simulink model "Alpha_Architecture"  (R2020b)
settings: Solver=VariableStepAuto  StartTime=0.0  StopTime=10.0  RelTol=1e-3
settings Model: DataDictionary=Alpha_ArchitectureDD_1.sldd  OrderedModelArguments=off  Creator=Josh_  LastModifiedBy=jbmic

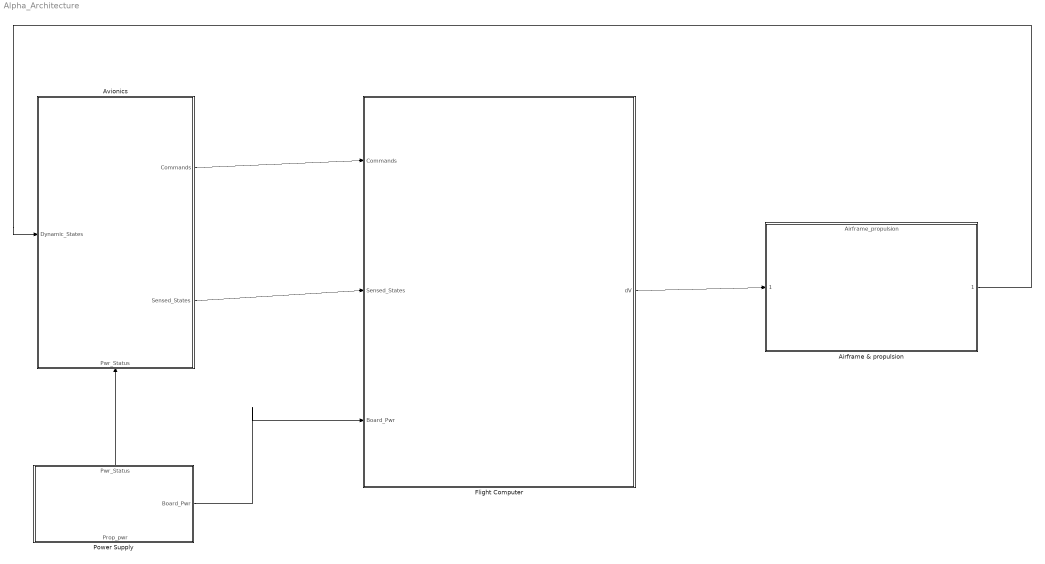
== system Alpha_Architecture ==
  Airframe & propulsion : ModelReference  ModelNameDialog=Airframe_propulsion  SimulationMode=Normal  ModelReferenceVersion=1.6
      settings: PortSchema="{\"entries\":[{\"content\":{\"headerSize\":38,\"margin\":15,\"minimumSpacing\":25,\"sides\":[{\"content\":{\"connectorIds\":[\"In1\"]},\"type\":\"ConnectorPlacement.EquallySpacedRectSide\",\"uuid\":\"5a96790b-1a4b-40de-9237-fa3ed351c29d\"},{\"content\":{\"connectorIds\":[\"Out1\"],\"side\":\"RIGHT\"},\"type\":\"ConnectorPlacement.EquallySpacedRectSide\",\"uuid\":\"65d1e4af-73af-4bc2-af7a-5ddd32d587af\"},{\"content\":{\"connectorIds\":[],\"side\":\"TOP\"},\"type\":\"ConnectorPlacement.EquallySpacedRectSide\",\"uuid\":\"28da9753-bb87-4f53-bc0d-c389ea44753a\"},{\"content\":{\"connectorIds\":[],\"side\":\"HIDDEN\"},\"type\":\"ConnectorPlacement.EquallySpacedRectSide\",\"uuid\":\"87ff2825-dc0e-4fcc-9b37-401c5c54474f\"}]},\"type\":\"ConnectorPlacement.EquallySpacedConnector\",\"uuid\":\"52ab39f8-c1eb-4e75-9fe9-b0e1857d3d38\"}],\"packageUris\":[\"http://schema.mathworks.com/mf0/Connector/R2020b\"],\"version\":\"1.0\"}"
  Avionics : Subsystem
      settings: PortSchema="{\"entries\":[{\"content\":{\"headerSize\":26,\"margin\":15,\"minimumSpacing\":25,\"sides\":[{\"content\":{\"connectorIds\":[\"In1\"]},\"type\":\"ConnectorPlacement.EquallySpacedRectSide\",\"uuid\":\"f0eb9bf2-bfee-4043-a89e-343ddad828c0\"},{\"content\":{\"connectorIds\":[\"Out1\",\"Out2\"],\"side\":\"RIGHT\"},\"type\":\"ConnectorPlacement.EquallySpacedRectSide\",\"uuid\":\"59a31ab0-f936-4a77-903b-0592fc94f50c\"},{\"content\":{\"connectorIds\":[],\"side\":\"TOP\"},\"type\":\"ConnectorPlacement.EquallySpacedRectSide\",\"uuid\":\"00c9f7f6-e065-44bb-91eb-10654e948fa4\"},{\"content\":{\"connectorIds\":[\"In2\"],\"side\":\"BOTTOM\"},\"type\":\"ConnectorPlacement.EquallySpacedRectSide\",\"uuid\":\"1c3b996c-1062-4d5b-bb11-b7de8dcf6a0a\"},{\"content\":{\"connectorIds\":[],\"side\":\"HIDDEN\"},\"type\":\"ConnectorPlacement.EquallySpacedRectSide\",\"uuid\":\"997c3d97-1a3e-4a81-af6b-83f3ee2d82f5\"}]},\"type\":\"ConnectorPlacement.EquallySpacedConnector\",\"uuid\":\"01157a40-eaa9-4a5a-9ab5-20d6af6643e5\"}],\"packageUris\":[\"http://schema.mathworks.com/mf0/Connector/R2020b\"],\"version\":\"1.0\"}"
  Flight Computer : Subsystem
      settings: PortSchema="{\"entries\":[{\"content\":{\"headerSize\":26,\"margin\":15,\"minimumSpacing\":25,\"sides\":[{\"content\":{\"connectorIds\":[\"In1\",\"In3\",\"In2\"]},\"type\":\"ConnectorPlacement.EquallySpacedRectSide\",\"uuid\":\"f0eb9bf2-bfee-4043-a89e-343ddad828c0\"},{\"content\":{\"connectorIds\":[\"Out1\"],\"side\":\"RIGHT\"},\"type\":\"ConnectorPlacement.EquallySpacedRectSide\",\"uuid\":\"59a31ab0-f936-4a77-903b-0592fc94f50c\"},{\"content\":{\"connectorIds\":[],\"side\":\"TOP\"},\"type\":\"ConnectorPlacement.EquallySpacedRectSide\",\"uuid\":\"00c9f7f6-e065-44bb-91eb-10654e948fa4\"},{\"content\":{\"connectorIds\":[],\"side\":\"BOTTOM\"},\"type\":\"ConnectorPlacement.EquallySpacedRectSide\",\"uuid\":\"e1a67c33-68ba-4a6b-a9bd-5a291173929b\"},{\"content\":{\"connectorIds\":[],\"side\":\"HIDDEN\"},\"type\":\"ConnectorPlacement.EquallySpacedRectSide\",\"uuid\":\"997c3d97-1a3e-4a81-af6b-83f3ee2d82f5\"}]},\"type\":\"ConnectorPlacement.EquallySpacedConnector\",\"uuid\":\"01157a40-eaa9-4a5a-9ab5-20d6af6643e5\"}],\"packageUris\":[\"http://schema.mathworks.com/mf0/Connector/R2020b\"],\"version\":\"1.0\"}"
  Power Supply : Subsystem
      settings: PortSchema="{\"entries\":[{\"content\":{\"headerSize\":26,\"margin\":15,\"minimumSpacing\":25,\"sides\":[{\"content\":{\"connectorIds\":[]},\"type\":\"ConnectorPlacement.EquallySpacedRectSide\",\"uuid\":\"f0eb9bf2-bfee-4043-a89e-343ddad828c0\"},{\"content\":{\"connectorIds\":[\"Out1\"],\"side\":\"RIGHT\"},\"type\":\"ConnectorPlacement.EquallySpacedRectSide\",\"uuid\":\"59a31ab0-f936-4a77-903b-0592fc94f50c\"},{\"content\":{\"connectorIds\":[\"Out3\"],\"side\":\"TOP\"},\"type\":\"ConnectorPlacement.EquallySpacedRectSide\",\"uuid\":\"00c9f7f6-e065-44bb-91eb-10654e948fa4\"},{\"content\":{\"connectorIds\":[\"Out2\"],\"side\":\"BOTTOM\"},\"type\":\"ConnectorPlacement.EquallySpacedRectSide\",\"uuid\":\"a7244861-68c9-40bc-a682-7b968120676e\"},{\"content\":{\"connectorIds\":[],\"side\":\"HIDDEN\"},\"type\":\"ConnectorPlacement.EquallySpacedRectSide\",\"uuid\":\"997c3d97-1a3e-4a81-af6b-83f3ee2d82f5\"}]},\"type\":\"ConnectorPlacement.EquallySpacedConnector\",\"uuid\":\"01157a40-eaa9-4a5a-9ab5-20d6af6643e5\"}],\"packageUris\":[\"http://schema.mathworks.com/mf0/Connector/R2020b\"],\"version\":\"1.0\"}"
  wires:
  Avionics/2(Sensed_States) -> Flight Computer/3(Sensed_States)
  Power Supply/3(Pwr_Status) -> Avionics/2(Pwr_Status)
  Avionics/1(Commands) -> Flight Computer/1(Commands)
  Power Supply/1(Board_Pwr) -> Flight Computer/2(Board_Pwr)
  Flight Computer/1(dV) -> Airframe & propulsion/1
  Airframe & propulsion/1 -> Avionics/1(Dynamic_States)

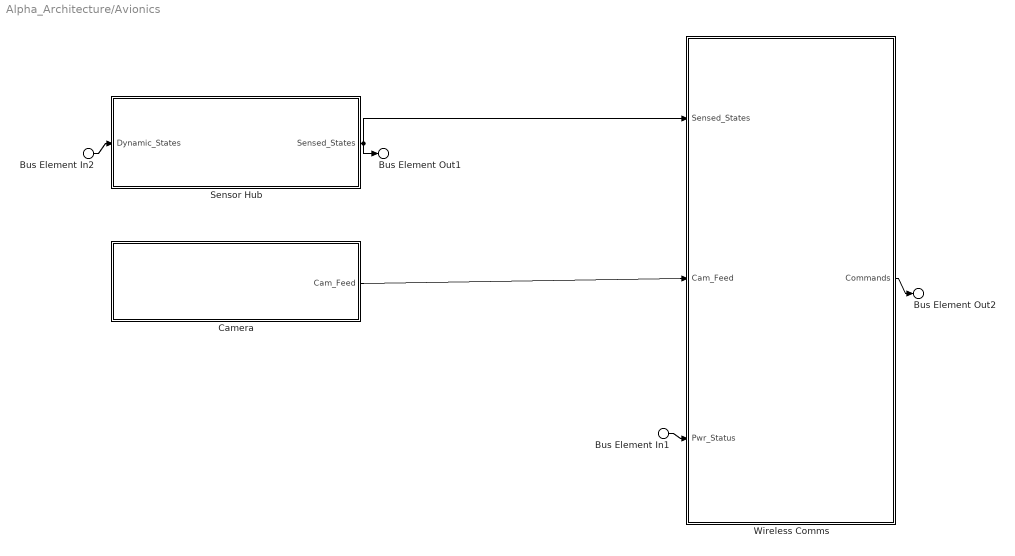
== system Alpha_Architecture/Avionics ==
  Bus Element In2 : Inport  PortName=Dynamic_States
  Bus Element In1 : Inport  Port=2  PortName=Pwr_Status
  Camera : Subsystem
      settings: PortSchema="{\"entries\":[{\"content\":{\"headerSize\":26,\"margin\":15,\"minimumSpacing\":25,\"sides\":[{\"content\":{\"connectorIds\":[]},\"type\":\"ConnectorPlacement.EquallySpacedRectSide\",\"uuid\":\"f0eb9bf2-bfee-4043-a89e-343ddad828c0\"},{\"content\":{\"connectorIds\":[\"Out1\"],\"side\":\"RIGHT\"},\"type\":\"ConnectorPlacement.EquallySpacedRectSide\",\"uuid\":\"59a31ab0-f936-4a77-903b-0592fc94f50c\"},{\"content\":{\"connectorIds\":[],\"side\":\"TOP\"},\"type\":\"ConnectorPlacement.EquallySpacedRectSide\",\"uuid\":\"00c9f7f6-e065-44bb-91eb-10654e948fa4\"},{\"content\":{\"connectorIds\":[],\"side\":\"HIDDEN\"},\"type\":\"ConnectorPlacement.EquallySpacedRectSide\",\"uuid\":\"997c3d97-1a3e-4a81-af6b-83f3ee2d82f5\"}]},\"type\":\"ConnectorPlacement.EquallySpacedConnector\",\"uuid\":\"01157a40-eaa9-4a5a-9ab5-20d6af6643e5\"}],\"packageUris\":[\"http://schema.mathworks.com/mf0/Connector/R2020b\"],\"version\":\"1.0\"}"
  Sensor Hub : Subsystem
      settings: PortSchema="{\"entries\":[{\"content\":{\"headerSize\":26,\"margin\":15,\"minimumSpacing\":25,\"sides\":[{\"content\":{\"connectorIds\":[\"In1\"]},\"type\":\"ConnectorPlacement.EquallySpacedRectSide\",\"uuid\":\"f0eb9bf2-bfee-4043-a89e-343ddad828c0\"},{\"content\":{\"connectorIds\":[\"Out1\"],\"side\":\"RIGHT\"},\"type\":\"ConnectorPlacement.EquallySpacedRectSide\",\"uuid\":\"59a31ab0-f936-4a77-903b-0592fc94f50c\"},{\"content\":{\"connectorIds\":[],\"side\":\"TOP\"},\"type\":\"ConnectorPlacement.EquallySpacedRectSide\",\"uuid\":\"00c9f7f6-e065-44bb-91eb-10654e948fa4\"},{\"content\":{\"connectorIds\":[],\"side\":\"HIDDEN\"},\"type\":\"ConnectorPlacement.EquallySpacedRectSide\",\"uuid\":\"997c3d97-1a3e-4a81-af6b-83f3ee2d82f5\"}]},\"type\":\"ConnectorPlacement.EquallySpacedConnector\",\"uuid\":\"01157a40-eaa9-4a5a-9ab5-20d6af6643e5\"}],\"packageUris\":[\"http://schema.mathworks.com/mf0/Connector/R2020b\"],\"version\":\"1.0\"}"
  Wireless Comms : Subsystem
      settings: PortSchema="{\"entries\":[{\"content\":{\"headerSize\":26,\"margin\":15,\"minimumSpacing\":25,\"sides\":[{\"content\":{\"connectorIds\":[\"In3\",\"In2\",\"In1\"]},\"type\":\"ConnectorPlacement.EquallySpacedRectSide\",\"uuid\":\"f0eb9bf2-bfee-4043-a89e-343ddad828c0\"},{\"content\":{\"connectorIds\":[\"Out1\"],\"side\":\"RIGHT\"},\"type\":\"ConnectorPlacement.EquallySpacedRectSide\",\"uuid\":\"59a31ab0-f936-4a77-903b-0592fc94f50c\"},{\"content\":{\"connectorIds\":[],\"side\":\"TOP\"},\"type\":\"ConnectorPlacement.EquallySpacedRectSide\",\"uuid\":\"00c9f7f6-e065-44bb-91eb-10654e948fa4\"},{\"content\":{\"connectorIds\":[],\"side\":\"HIDDEN\"},\"type\":\"ConnectorPlacement.EquallySpacedRectSide\",\"uuid\":\"997c3d97-1a3e-4a81-af6b-83f3ee2d82f5\"}]},\"type\":\"ConnectorPlacement.EquallySpacedConnector\",\"uuid\":\"01157a40-eaa9-4a5a-9ab5-20d6af6643e5\"}],\"packageUris\":[\"http://schema.mathworks.com/mf0/Connector/R2020b\"],\"version\":\"1.0\"}"
  Bus Element Out2 : Outport  PortName=Commands
  Bus Element Out1 : Outport  Port=2  PortName=Sensed_States
  wires:
  Camera/1(Cam_Feed) -> Wireless Comms/2(Cam_Feed)
  Sensor Hub/1(Sensed_States) -> Wireless Comms/3(Sensed_States), Bus Element Out1/1
  Bus Element In1/1 -> Wireless Comms/1(Pwr_Status)
  Wireless Comms/1(Commands) -> Bus Element Out2/1
  Bus Element In2/1 -> Sensor Hub/1(Dynamic_States)

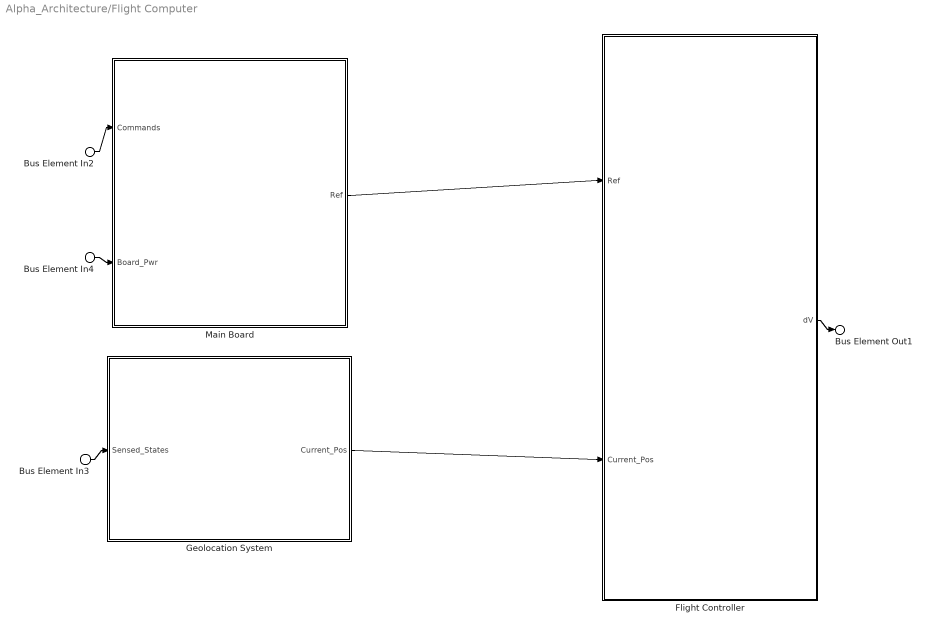
== system Alpha_Architecture/Flight Computer ==
  Bus Element In2 : Inport  PortName=Commands
  Bus Element In4 : Inport  Port=2  PortName=Board_Pwr
  Bus Element In3 : Inport  Port=3  PortName=Sensed_States
  Flight Controller : Subsystem
      settings: PortSchema="{\"entries\":[{\"content\":{\"headerSize\":26,\"margin\":15,\"minimumSpacing\":25,\"sides\":[{\"content\":{\"connectorIds\":[\"In1\",\"In2\"]},\"type\":\"ConnectorPlacement.EquallySpacedRectSide\",\"uuid\":\"f0eb9bf2-bfee-4043-a89e-343ddad828c0\"},{\"content\":{\"connectorIds\":[\"Out1\"],\"side\":\"RIGHT\"},\"type\":\"ConnectorPlacement.EquallySpacedRectSide\",\"uuid\":\"59a31ab0-f936-4a77-903b-0592fc94f50c\"},{\"content\":{\"connectorIds\":[],\"side\":\"TOP\"},\"type\":\"ConnectorPlacement.EquallySpacedRectSide\",\"uuid\":\"00c9f7f6-e065-44bb-91eb-10654e948fa4\"},{\"content\":{\"connectorIds\":[],\"side\":\"BOTTOM\"},\"type\":\"ConnectorPlacement.EquallySpacedRectSide\",\"uuid\":\"961fc88a-8781-4ec4-8a6a-b42b081babd4\"},{\"content\":{\"connectorIds\":[],\"side\":\"HIDDEN\"},\"type\":\"ConnectorPlacement.EquallySpacedRectSide\",\"uuid\":\"997c3d97-1a3e-4a81-af6b-83f3ee2d82f5\"}]},\"type\":\"ConnectorPlacement.EquallySpacedConnector\",\"uuid\":\"01157a40-eaa9-4a5a-9ab5-20d6af6643e5\"}],\"packageUris\":[\"http://schema.mathworks.com/mf0/Connector/R2020b\"],\"version\":\"1.0\"}"
  Geolocation System : Subsystem
      settings: PortSchema="{\"entries\":[{\"content\":{\"headerSize\":26,\"margin\":15,\"minimumSpacing\":25,\"sides\":[{\"content\":{\"connectorIds\":[\"In1\"]},\"type\":\"ConnectorPlacement.EquallySpacedRectSide\",\"uuid\":\"f0eb9bf2-bfee-4043-a89e-343ddad828c0\"},{\"content\":{\"connectorIds\":[\"Out1\"],\"side\":\"RIGHT\"},\"type\":\"ConnectorPlacement.EquallySpacedRectSide\",\"uuid\":\"59a31ab0-f936-4a77-903b-0592fc94f50c\"},{\"content\":{\"connectorIds\":[],\"side\":\"TOP\"},\"type\":\"ConnectorPlacement.EquallySpacedRectSide\",\"uuid\":\"00c9f7f6-e065-44bb-91eb-10654e948fa4\"},{\"content\":{\"connectorIds\":[],\"side\":\"HIDDEN\"},\"type\":\"ConnectorPlacement.EquallySpacedRectSide\",\"uuid\":\"997c3d97-1a3e-4a81-af6b-83f3ee2d82f5\"}]},\"type\":\"ConnectorPlacement.EquallySpacedConnector\",\"uuid\":\"01157a40-eaa9-4a5a-9ab5-20d6af6643e5\"}],\"packageUris\":[\"http://schema.mathworks.com/mf0/Connector/R2020b\"],\"version\":\"1.0\"}"
  Main Board : Subsystem
      settings: PortSchema="{\"entries\":[{\"content\":{\"headerSize\":26,\"margin\":15,\"minimumSpacing\":25,\"sides\":[{\"content\":{\"connectorIds\":[\"In2\",\"In1\"]},\"type\":\"ConnectorPlacement.EquallySpacedRectSide\",\"uuid\":\"f0eb9bf2-bfee-4043-a89e-343ddad828c0\"},{\"content\":{\"connectorIds\":[\"Out1\"],\"side\":\"RIGHT\"},\"type\":\"ConnectorPlacement.EquallySpacedRectSide\",\"uuid\":\"59a31ab0-f936-4a77-903b-0592fc94f50c\"},{\"content\":{\"connectorIds\":[],\"side\":\"TOP\"},\"type\":\"ConnectorPlacement.EquallySpacedRectSide\",\"uuid\":\"00c9f7f6-e065-44bb-91eb-10654e948fa4\"},{\"content\":{\"connectorIds\":[],\"side\":\"BOTTOM\"},\"type\":\"ConnectorPlacement.EquallySpacedRectSide\",\"uuid\":\"d3df3a47-29ff-4127-ba11-03dc604beefc\"},{\"content\":{\"connectorIds\":[],\"side\":\"HIDDEN\"},\"type\":\"ConnectorPlacement.EquallySpacedRectSide\",\"uuid\":\"997c3d97-1a3e-4a81-af6b-83f3ee2d82f5\"}]},\"type\":\"ConnectorPlacement.EquallySpacedConnector\",\"uuid\":\"01157a40-eaa9-4a5a-9ab5-20d6af6643e5\"}],\"packageUris\":[\"http://schema.mathworks.com/mf0/Connector/R2020b\"],\"version\":\"1.0\"}"
  Bus Element Out1 : Outport  PortName=dV
  wires:
  Flight Controller/1(dV) -> Bus Element Out1/1
  Main Board/1(Ref) -> Flight Controller/1(Ref)
  Bus Element In2/1 -> Main Board/2(Commands)
  Bus Element In4/1 -> Main Board/1(Board_Pwr)
  Bus Element In3/1 -> Geolocation System/1(Sensed_States)
  Geolocation System/1(Current_Pos) -> Flight Controller/2(Current_Pos)

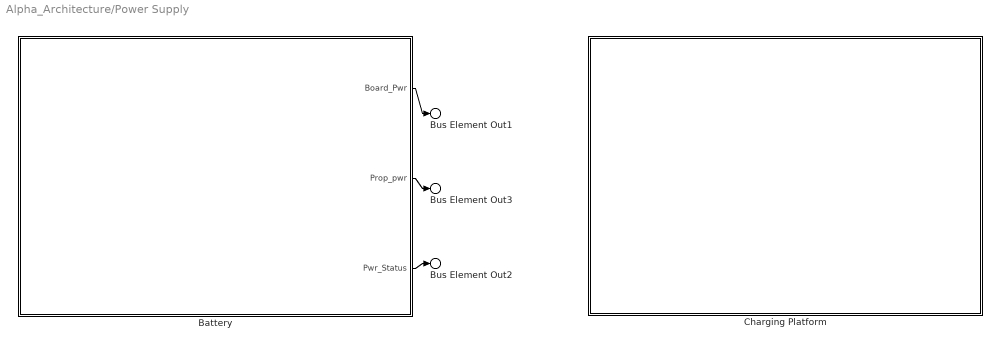
== system Alpha_Architecture/Power Supply ==
  Battery : Subsystem
      settings: PortSchema="{\"entries\":[{\"content\":{\"headerSize\":26,\"margin\":15,\"minimumSpacing\":25,\"sides\":[{\"content\":{\"connectorIds\":[]},\"type\":\"ConnectorPlacement.EquallySpacedRectSide\",\"uuid\":\"f0eb9bf2-bfee-4043-a89e-343ddad828c0\"},{\"content\":{\"connectorIds\":[\"Out1\",\"Out2\",\"Out3\"],\"side\":\"RIGHT\"},\"type\":\"ConnectorPlacement.EquallySpacedRectSide\",\"uuid\":\"59a31ab0-f936-4a77-903b-0592fc94f50c\"},{\"content\":{\"connectorIds\":[],\"side\":\"TOP\"},\"type\":\"ConnectorPlacement.EquallySpacedRectSide\",\"uuid\":\"00c9f7f6-e065-44bb-91eb-10654e948fa4\"},{\"content\":{\"connectorIds\":[],\"side\":\"HIDDEN\"},\"type\":\"ConnectorPlacement.EquallySpacedRectSide\",\"uuid\":\"997c3d97-1a3e-4a81-af6b-83f3ee2d82f5\"}]},\"type\":\"ConnectorPlacement.EquallySpacedConnector\",\"uuid\":\"01157a40-eaa9-4a5a-9ab5-20d6af6643e5\"}],\"packageUris\":[\"http://schema.mathworks.com/mf0/Connector/R2020b\"],\"version\":\"1.0\"}"
  Charging Platform : Subsystem
      settings: PortSchema="{\"entries\":[{\"content\":{\"headerSize\":26,\"margin\":15,\"minimumSpacing\":25,\"sides\":[{\"content\":{\"connectorIds\":[]},\"type\":\"ConnectorPlacement.EquallySpacedRectSide\",\"uuid\":\"f0eb9bf2-bfee-4043-a89e-343ddad828c0\"},{\"content\":{\"connectorIds\":[],\"side\":\"RIGHT\"},\"type\":\"ConnectorPlacement.EquallySpacedRectSide\",\"uuid\":\"59a31ab0-f936-4a77-903b-0592fc94f50c\"},{\"content\":{\"connectorIds\":[],\"side\":\"TOP\"},\"type\":\"ConnectorPlacement.EquallySpacedRectSide\",\"uuid\":\"00c9f7f6-e065-44bb-91eb-10654e948fa4\"},{\"content\":{\"connectorIds\":[],\"side\":\"HIDDEN\"},\"type\":\"ConnectorPlacement.EquallySpacedRectSide\",\"uuid\":\"997c3d97-1a3e-4a81-af6b-83f3ee2d82f5\"}]},\"type\":\"ConnectorPlacement.EquallySpacedConnector\",\"uuid\":\"01157a40-eaa9-4a5a-9ab5-20d6af6643e5\"}],\"packageUris\":[\"http://schema.mathworks.com/mf0/Connector/R2020b\"],\"version\":\"1.0\"}"
  Bus Element Out1 : Outport  PortName=Board_Pwr
  Bus Element Out3 : Outport  Port=2  PortName=Prop_pwr
  Bus Element Out2 : Outport  Port=3  PortName=Pwr_Status
  wires:
  Battery/3(Pwr_Status) -> Bus Element Out2/1
  Battery/1(Board_Pwr) -> Bus Element Out1/1
  Battery/2(Prop_pwr) -> Bus Element Out3/1

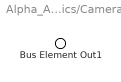
== system Alpha_Architecture/Avionics/Camera ==
  Bus Element Out1 : Outport  PortName=Cam_Feed

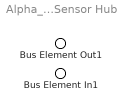
== system Alpha_Architecture/Avionics/Sensor Hub ==
  Bus Element In1 : Inport  PortName=Dynamic_States
  Bus Element Out1 : Outport  PortName=Sensed_States

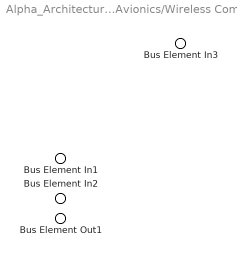
== system Alpha_Architecture/Avionics/Wireless Comms ==
  Bus Element In3 : Inport  PortName=Pwr_Status
  Bus Element In1 : Inport  Port=2  PortName=Cam_Feed
  Bus Element In2 : Inport  Port=3  PortName=Sensed_States
  Bus Element Out1 : Outport  PortName=Commands

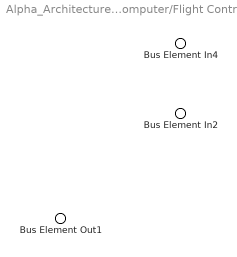
== system Alpha_Architecture/Flight Computer/Flight Controller ==
  Bus Element In4 : Inport  PortName=Ref
  Bus Element In2 : Inport  Port=2  PortName=Current_Pos
  Bus Element Out1 : Outport  PortName=dV

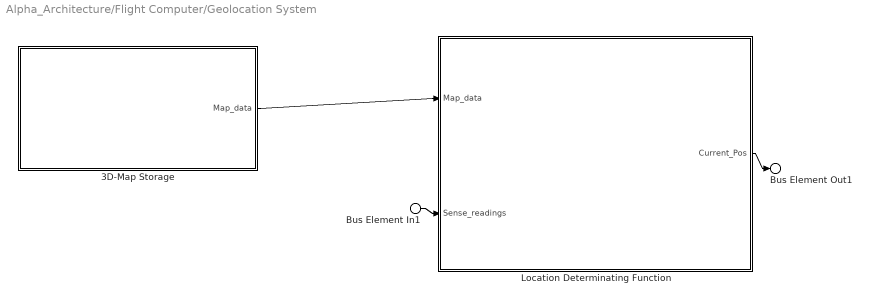
== system Alpha_Architecture/Flight Computer/Geolocation System ==
  Bus Element In1 : Inport  PortName=Sensed_States
  3D-Map Storage : Subsystem
      settings: PortSchema="{\"entries\":[{\"content\":{\"headerSize\":26,\"margin\":15,\"minimumSpacing\":25,\"sides\":[{\"content\":{\"connectorIds\":[]},\"type\":\"ConnectorPlacement.EquallySpacedRectSide\",\"uuid\":\"f0eb9bf2-bfee-4043-a89e-343ddad828c0\"},{\"content\":{\"connectorIds\":[\"Out1\"],\"side\":\"RIGHT\"},\"type\":\"ConnectorPlacement.EquallySpacedRectSide\",\"uuid\":\"59a31ab0-f936-4a77-903b-0592fc94f50c\"},{\"content\":{\"connectorIds\":[],\"side\":\"TOP\"},\"type\":\"ConnectorPlacement.EquallySpacedRectSide\",\"uuid\":\"00c9f7f6-e065-44bb-91eb-10654e948fa4\"},{\"content\":{\"connectorIds\":[],\"side\":\"HIDDEN\"},\"type\":\"ConnectorPlacement.EquallySpacedRectSide\",\"uuid\":\"997c3d97-1a3e-4a81-af6b-83f3ee2d82f5\"}]},\"type\":\"ConnectorPlacement.EquallySpacedConnector\",\"uuid\":\"01157a40-eaa9-4a5a-9ab5-20d6af6643e5\"}],\"packageUris\":[\"http://schema.mathworks.com/mf0/Connector/R2020b\"],\"version\":\"1.0\"}"
  Location Determinating Function : Subsystem
      settings: PortSchema="{\"entries\":[{\"content\":{\"headerSize\":26,\"margin\":15,\"minimumSpacing\":25,\"sides\":[{\"content\":{\"connectorIds\":[\"In1\",\"In2\"]},\"type\":\"ConnectorPlacement.EquallySpacedRectSide\",\"uuid\":\"f0eb9bf2-bfee-4043-a89e-343ddad828c0\"},{\"content\":{\"connectorIds\":[\"Out1\"],\"side\":\"RIGHT\"},\"type\":\"ConnectorPlacement.EquallySpacedRectSide\",\"uuid\":\"59a31ab0-f936-4a77-903b-0592fc94f50c\"},{\"content\":{\"connectorIds\":[],\"side\":\"TOP\"},\"type\":\"ConnectorPlacement.EquallySpacedRectSide\",\"uuid\":\"00c9f7f6-e065-44bb-91eb-10654e948fa4\"},{\"content\":{\"connectorIds\":[],\"side\":\"HIDDEN\"},\"type\":\"ConnectorPlacement.EquallySpacedRectSide\",\"uuid\":\"997c3d97-1a3e-4a81-af6b-83f3ee2d82f5\"}]},\"type\":\"ConnectorPlacement.EquallySpacedConnector\",\"uuid\":\"01157a40-eaa9-4a5a-9ab5-20d6af6643e5\"}],\"packageUris\":[\"http://schema.mathworks.com/mf0/Connector/R2020b\"],\"version\":\"1.0\"}"
  Bus Element Out1 : Outport  PortName=Current_Pos
  wires:
  3D-Map Storage/1(Map_data) -> Location Determinating Function/1(Map_data)
  Bus Element In1/1 -> Location Determinating Function/2(Sense_readings)
  Location Determinating Function/1(Current_Pos) -> Bus Element Out1/1

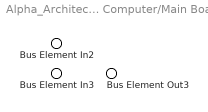
== system Alpha_Architecture/Flight Computer/Main Board ==
  Bus Element In3 : Inport  PortName=Board_Pwr
  Bus Element In2 : Inport  Port=2  PortName=Commands
  Bus Element Out3 : Outport  PortName=Ref

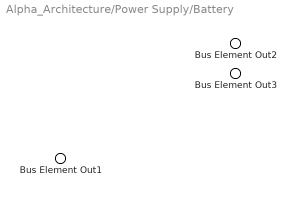
== system Alpha_Architecture/Power Supply/Battery ==
  Bus Element Out2 : Outport  PortName=Board_Pwr
  Bus Element Out3 : Outport  Port=2  PortName=Prop_pwr
  Bus Element Out1 : Outport  Port=3  PortName=Pwr_Status

== system Alpha_Architecture/Power Supply/Charging Platform ==

== system Alpha_Architecture/Flight Computer/Geolocation System/3D-Map Storage ==
  Bus Element Out1 : Outport  PortName=Map_data

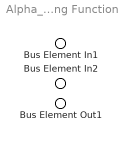
== system Alpha_Architecture/Flight Computer/Geolocation System/Location Determinating Function ==
  Bus Element In1 : Inport  PortName=Map_data
  Bus Element In2 : Inport  Port=2  PortName=Sense_readings
  Bus Element Out1 : Outport  PortName=Current_Pos
